simulink model "bike_system_o"  (R2018b)
settings: Solver=VariableStepAuto  StartTime=0.0  StopTime=10.0  RelTol=1e-3
values from neighbouring files (symbols this model uses):
  A = [0 g/h;1 0]    [setup.m]
  B = (a*v/(b*h))*[1; v/a]    [setup.m]
  C = [1 0;0 1]    [setup.m]
  Ts = 0.04    [setup.m]
undefined symbols (not defined in the file or in its folder): Kd
settings Model: Creator=jonas  LastModifiedBy=maximef
settings DataIOCC: ReturnWorkspaceOutputs=on

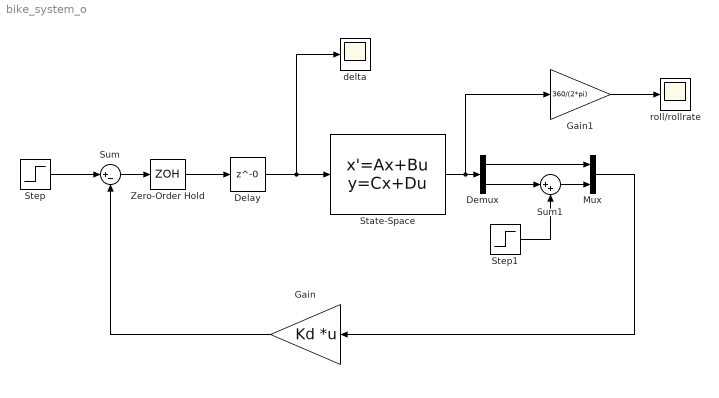
== system bike_system_o ==
  Delay : Delay  DelayLength=0  InitialCondition=0  SampleTime=Ts
  Demux : Demux  Outputs=2
  Gain : Gain  Gain=Kd  Multiplication=Matrix(K*u) (u vector)
  Gain1 : Gain  Gain=360/(2*pi)
  Mux : Mux  Inputs=2
  State-Space : StateSpace  A=A  B=B  C=C  D=[0 ;0]  InitialCondition=0  ContinuousStateAttributes='roll'
  Step : Step  Time=5  After=5*2*pi/360  SampleTime=0
  Step1 : Step  After=2*2*pi/360  SampleTime=0
  Sum : Sum  Inputs=|+-
  Sum1 : Sum  Inputs=|++
  Zero-Order Hold : ZeroOrderHold  SampleTime=Ts
  delta : Scope
  roll/rollrate : Scope
  wires:
  Zero-Order Hold/1 -> Delay/1
  Sum/1 -> Zero-Order Hold/1
  Gain/1 -> Sum/2
  Step/1 -> Sum/1
  State-Space/1 -> Gain1/1, Demux/1
  Demux/2 -> Sum1/1
  Step1/1 -> Sum1/2
  Mux/1 -> Gain/1
  Demux/1 -> Mux/1
  Sum1/1 -> Mux/2
  Gain1/1 -> roll/rollrate/1
  Delay/1 -> State-Space/1, delta/1
